simulink model "simu11"  (R2016b)
settings: Solver=VariableStepAuto  StartTime=0.0  StopTime=10.0  RelTol=1e-3
libraries: ArbolFallosLIB x185
settings Model: Creator=inmaculadacoronaperez  LastModifiedBy=josed

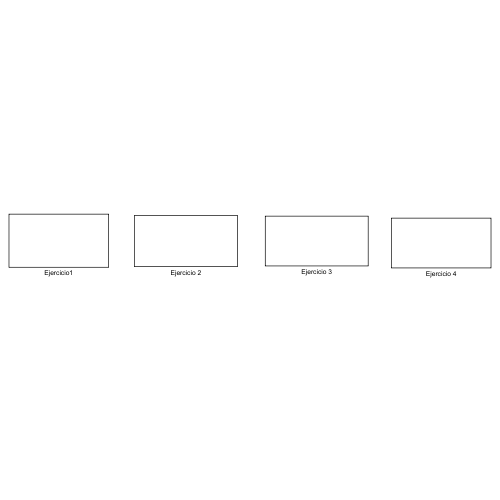
[thumbnail: Simulink's stored preview of the top-level diagram]
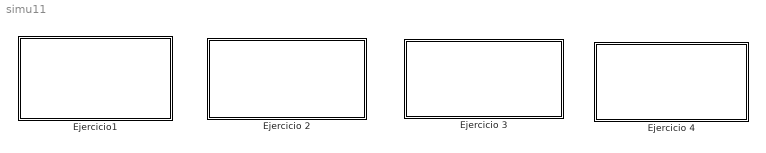
== system simu11 ==
  "Ejercicio 2 " : Subsystem
  "Ejercicio 3 " : Subsystem
  Ejercicio 4 : Subsystem
  "Ejercicio1 " : Subsystem

== system simu11/Ejercicio 2  ==
  Apartado b : Subsystem
  Apartado c : Subsystem
  wires:
  Apartado b/1(Out1) -> [s2_apb]
  [s2_apb] -> Apartado c/1(In1)

== system simu11/Ejercicio 3  ==
  APARTADO A : Subsystem
  Subsystem : Subsystem
  wires:
  APARTADO A/1(Out1) -> [lambda_elevador]
  [lambda_elevador] -> Subsystem/1(In1)

== system simu11/Ejercicio 4 ==
  APARTADO B : Subsystem
  APARTADO C : Subsystem
  APARTADO D : Subsystem
  APARTADO E : Subsystem

== system simu11/Ejercicio1  ==
  Ejercicio 1 a) : Subsystem
  Ejercicio 1 b) : Subsystem

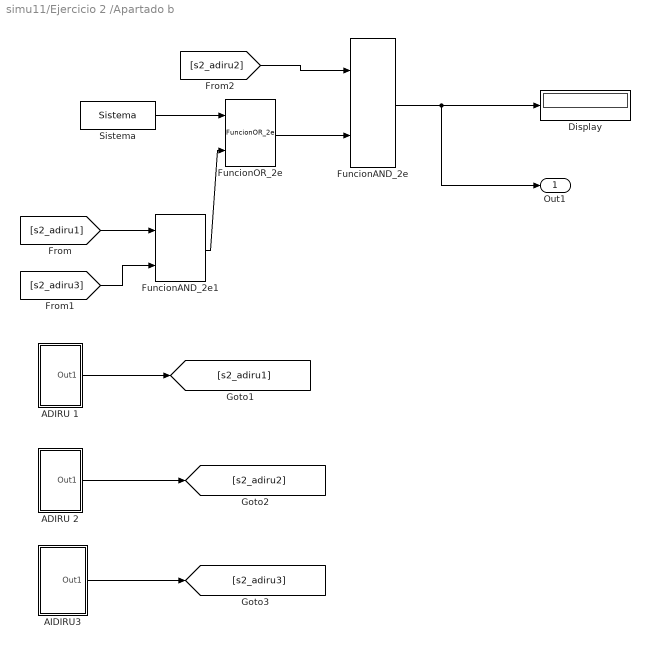
== system simu11/Ejercicio 2 /Apartado b ==
  ADIRU 1 : Subsystem
  ADIRU 2 : Subsystem
  AIDIRU3 : Subsystem
  Display : Display
  FuncionAND_2e : ArbolFallosLIB/FuncionAND_2e  SystemSampleTime=-1  Latency=0  AutoFrameSizeCalculation=off
  FuncionAND_2e1 : ArbolFallosLIB/FuncionAND_2e  SystemSampleTime=-1  Latency=0  AutoFrameSizeCalculation=off
  FuncionOR_2e : ArbolFallosLIB/FuncionOR_2e  SystemSampleTime=-1  Latency=0  AutoFrameSizeCalculation=off
  Sistema : ArbolFallosLIB/Sistema  sistema='CAPT TAT'  lambda=5e-04
  Out1 : Outport
  wires:
  [s2_adiru1] -> FuncionAND_2e1/1
  Sistema/1 -> FuncionOR_2e/1
  FuncionAND_2e/1 -> Out1/1, Display/1
  [s2_adiru3] -> FuncionAND_2e1/2
  FuncionAND_2e1/1 -> FuncionOR_2e/2
  FuncionOR_2e/1 -> FuncionAND_2e/2
  [s2_adiru2] -> FuncionAND_2e/1
  ADIRU 1/1(Out1) -> [s2_adiru1]
  ADIRU 2/1(Out1) -> [s2_adiru2]
  AIDIRU3/1(Out1) -> [s2_adiru3]

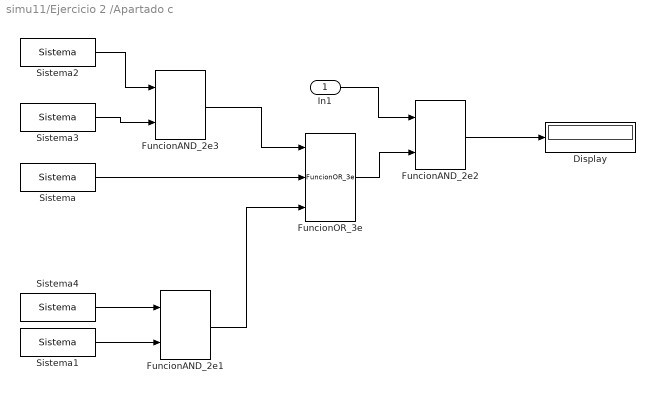
== system simu11/Ejercicio 2 /Apartado c ==
  In1 : Inport
  Display : Display
  FuncionAND_2e1 : ArbolFallosLIB/FuncionAND_2e  SystemSampleTime=-1  Latency=0  AutoFrameSizeCalculation=off
  FuncionAND_2e2 : ArbolFallosLIB/FuncionAND_2e  SystemSampleTime=-1  Latency=0  AutoFrameSizeCalculation=off
  FuncionAND_2e3 : ArbolFallosLIB/FuncionAND_2e  SystemSampleTime=-1  Latency=0  AutoFrameSizeCalculation=off
  FuncionOR_3e : ArbolFallosLIB/FuncionOR_3e  SystemSampleTime=-1  Latency=0  AutoFrameSizeCalculation=off
  Sistema : ArbolFallosLIB/Sistema  sistema='PITOT STBY'  lambda=2e-03
  Sistema1 : ArbolFallosLIB/Sistema  sistema='STATIC STBY'  lambda=1.5e-03
  Sistema2 : ArbolFallosLIB/Sistema  sistema='STBY ASI'  lambda=5e-03
  Sistema3 : ArbolFallosLIB/Sistema  sistema='STBY ALTI'  lambda=5e-03
  Sistema4 : ArbolFallosLIB/Sistema  sistema='STATIC STBY'  lambda=1.5e-03
  wires:
  Sistema/1 -> FuncionOR_3e/2
  Sistema4/1 -> FuncionAND_2e1/1
  Sistema1/1 -> FuncionAND_2e1/2
  FuncionAND_2e1/1 -> FuncionOR_3e/3
  FuncionOR_3e/1 -> FuncionAND_2e2/2
  Sistema2/1 -> FuncionAND_2e3/1
  Sistema3/1 -> FuncionAND_2e3/2
  FuncionAND_2e3/1 -> FuncionOR_3e/1
  In1/1 -> FuncionAND_2e2/1
  FuncionAND_2e2/1 -> Display/1

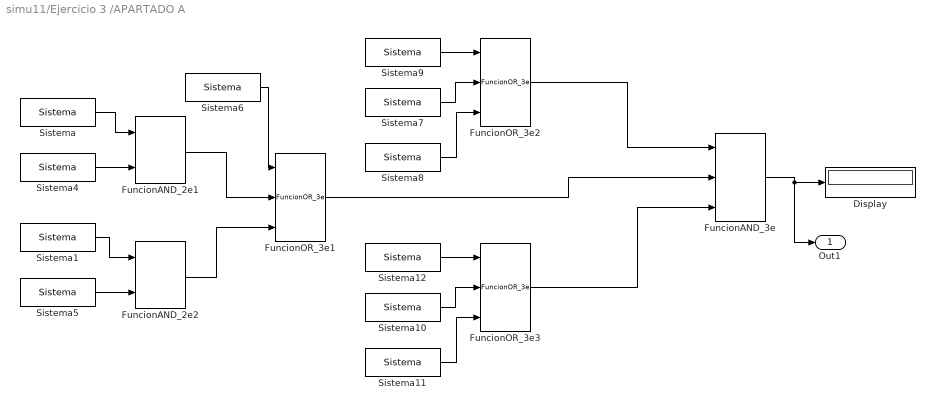
== system simu11/Ejercicio 3 /APARTADO A ==
  Display : Display
  FuncionAND_2e1 : ArbolFallosLIB/FuncionAND_2e  SystemSampleTime=-1  Latency=0  AutoFrameSizeCalculation=off
  FuncionAND_2e2 : ArbolFallosLIB/FuncionAND_2e  SystemSampleTime=-1  Latency=0  AutoFrameSizeCalculation=off
  FuncionAND_3e : ArbolFallosLIB/FuncionAND_3e  SystemSampleTime=-1  Latency=0  AutoFrameSizeCalculation=off
  FuncionOR_3e1 : ArbolFallosLIB/FuncionOR_3e  SystemSampleTime=-1  Latency=0  AutoFrameSizeCalculation=off
  FuncionOR_3e2 : ArbolFallosLIB/FuncionOR_3e  SystemSampleTime=-1  Latency=0  AutoFrameSizeCalculation=off
  FuncionOR_3e3 : ArbolFallosLIB/FuncionOR_3e  SystemSampleTime=-1  Latency=0  AutoFrameSizeCalculation=off
  Sistema : ArbolFallosLIB/Sistema  sistema='ACT RHO'  lambda=2.5e-04
  Sistema1 : ArbolFallosLIB/Sistema  sistema='Databus 2'  lambda=1e-8
  Sistema10 : ArbolFallosLIB/Sistema  sistema='HYD G'  lambda=2e-4
  Sistema11 : ArbolFallosLIB/Sistema  sistema='Databus 4'  lambda=1e-8
  Sistema12 : ArbolFallosLIB/Sistema  sistema='ACTUADOR LHI'  lambda=2.5e-04
  Sistema4 : ArbolFallosLIB/Sistema  sistema='ACT LHO'  lambda=2.5e-04
  Sistema5 : ArbolFallosLIB/Sistema  sistema='Databus 3'  lambda=1e-8
  Sistema6 : ArbolFallosLIB/Sistema  sistema='HYD B'  lambda=2e-4
  Sistema7 : ArbolFallosLIB/Sistema  sistema='HYD Y'  lambda=2e-4
  Sistema8 : ArbolFallosLIB/Sistema  sistema='Databus 1'  lambda=1e-8
  Sistema9 : ArbolFallosLIB/Sistema  sistema='ACTUADOR RHI'  lambda=2.5e-04
  Out1 : Outport
  wires:
  FuncionAND_3e/1 -> Display/1, Out1/1
  FuncionAND_2e2/1 -> FuncionOR_3e1/3
  Sistema5/1 -> FuncionAND_2e2/2
  Sistema9/1 -> FuncionOR_3e2/1
  Sistema/1 -> FuncionAND_2e1/1
  Sistema4/1 -> FuncionAND_2e1/2
  Sistema8/1 -> FuncionOR_3e2/3
  FuncionOR_3e3/1 -> FuncionAND_3e/3
  Sistema7/1 -> FuncionOR_3e2/2
  FuncionOR_3e2/1 -> FuncionAND_3e/1
  Sistema12/1 -> FuncionOR_3e3/1
  Sistema10/1 -> FuncionOR_3e3/2
  Sistema11/1 -> FuncionOR_3e3/3
  FuncionOR_3e1/1 -> FuncionAND_3e/2
  FuncionAND_2e1/1 -> FuncionOR_3e1/2
  Sistema1/1 -> FuncionAND_2e2/1
  Sistema6/1 -> FuncionOR_3e1/1

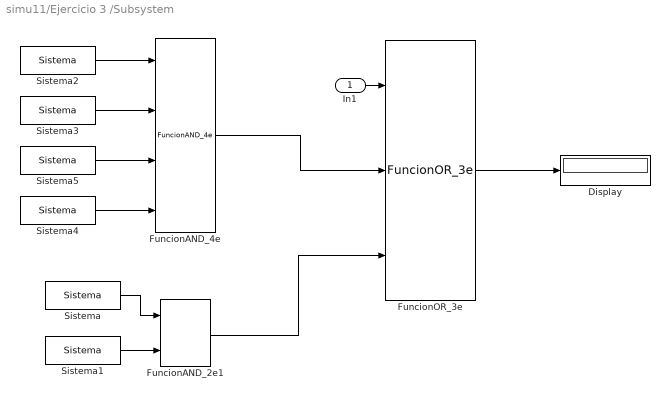
== system simu11/Ejercicio 3 /Subsystem ==
  In1 : Inport
  Display : Display
  FuncionAND_2e1 : ArbolFallosLIB/FuncionAND_2e  SystemSampleTime=-1  Latency=0  AutoFrameSizeCalculation=off
  FuncionAND_4e : ArbolFallosLIB/FuncionAND_4e  SystemSampleTime=-1  Latency=0  AutoFrameSizeCalculation=off
  FuncionOR_3e : ArbolFallosLIB/FuncionOR_3e  SystemSampleTime=-1  Latency=0  AutoFrameSizeCalculation=off
  Sistema : ArbolFallosLIB/Sistema  sistema='STICK CAPT'  lambda=2e-06
  Sistema1 : ArbolFallosLIB/Sistema  sistema='STICK F/O'  lambda=2e-06
  Sistema2 : ArbolFallosLIB/Sistema  sistema='ELAC 1'  lambda=1e-04
  Sistema3 : ArbolFallosLIB/Sistema  sistema='ELAC 2'  lambda=1e-04
  Sistema4 : ArbolFallosLIB/Sistema  sistema='ELAC 4'  lambda=1e-04
  Sistema5 : ArbolFallosLIB/Sistema  sistema='ELAC 3'  lambda=1e-04
  wires:
  Sistema3/1 -> FuncionAND_4e/2
  Sistema/1 -> FuncionAND_2e1/1
  FuncionAND_2e1/1 -> FuncionOR_3e/3
  Sistema1/1 -> FuncionAND_2e1/2
  Sistema4/1 -> FuncionAND_4e/4
  Sistema2/1 -> FuncionAND_4e/1
  FuncionAND_4e/1 -> FuncionOR_3e/2
  In1/1 -> FuncionOR_3e/1
  Sistema5/1 -> FuncionAND_4e/3
  FuncionOR_3e/1 -> Display/1

== system simu11/Ejercicio 4/APARTADO B ==
  Display : Display
  FuncionOR_2e1 : ArbolFallosLIB/FuncionOR_2e  SystemSampleTime=-1  Latency=0  AutoFrameSizeCalculation=off
  FuncionOR_2e2 : ArbolFallosLIB/FuncionOR_2e  SystemSampleTime=-1  Latency=0  AutoFrameSizeCalculation=off
  FuncionOR_2e3 : ArbolFallosLIB/FuncionOR_2e  SystemSampleTime=-1  Latency=0  AutoFrameSizeCalculation=off
  Sistema : ArbolFallosLIB/Sistema  sistema='COM'  lambda=5e-4
  Sistema1 : ArbolFallosLIB/Sistema  sistema='MON'  lambda=7e-4
  Sistema2 : ArbolFallosLIB/Sistema  sistema='COM'  lambda=5e-4
  Sistema3 : ArbolFallosLIB/Sistema  sistema='MON'  lambda=7e-4
  wires:
  FuncionOR_2e3/1 -> Display/1
  Sistema1/1 -> FuncionOR_2e1/2
  Sistema/1 -> FuncionOR_2e1/1
  Sistema3/1 -> FuncionOR_2e2/2
  Sistema2/1 -> FuncionOR_2e2/1
  FuncionOR_2e1/1 -> FuncionOR_2e3/1
  FuncionOR_2e2/1 -> FuncionOR_2e3/2

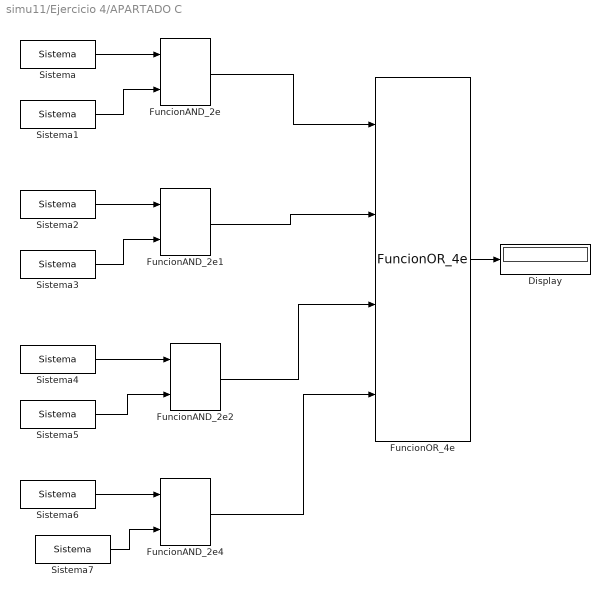
== system simu11/Ejercicio 4/APARTADO C ==
  Display : Display
  FuncionAND_2e{,1..2,4} (4 alike) : ArbolFallosLIB/FuncionAND_2e  SystemSampleTime=-1  Latency=0  AutoFrameSizeCalculation=off
  FuncionOR_4e : ArbolFallosLIB/FuncionOR_4e  SystemSampleTime=-1  Latency=0  AutoFrameSizeCalculation=off
  Sistema : ArbolFallosLIB/Sistema  sistema='COM_A'  lambda=5e-4
  Sistema1 : ArbolFallosLIB/Sistema  sistema='COM_B'  lambda=5e-4
  Sistema2 : ArbolFallosLIB/Sistema  sistema='MON_A'  lambda=7e-4
  Sistema3 : ArbolFallosLIB/Sistema  sistema='MON_B'  lambda=7e-4
  Sistema4 : ArbolFallosLIB/Sistema  sistema='COM_A'  lambda=5e-4
  Sistema5 : ArbolFallosLIB/Sistema  sistema='MON_B'  lambda=7e-4
  Sistema6 : ArbolFallosLIB/Sistema  sistema='MON_A'  lambda=7e-4
  Sistema7 : ArbolFallosLIB/Sistema  sistema='COM_B'  lambda=5e-4
  wires:
  Sistema1/1 -> FuncionAND_2e/2
  Sistema/1 -> FuncionAND_2e/1
  Sistema6/1 -> FuncionAND_2e4/1
  Sistema7/1 -> FuncionAND_2e4/2
  FuncionAND_2e1/1 -> FuncionOR_4e/2
  FuncionAND_2e4/1 -> FuncionOR_4e/4
  Sistema5/1 -> FuncionAND_2e2/2
  Sistema2/1 -> FuncionAND_2e1/1
  Sistema3/1 -> FuncionAND_2e1/2
  FuncionAND_2e/1 -> FuncionOR_4e/1
  FuncionOR_4e/1 -> Display/1
  Sistema4/1 -> FuncionAND_2e2/1
  FuncionAND_2e2/1 -> FuncionOR_4e/3

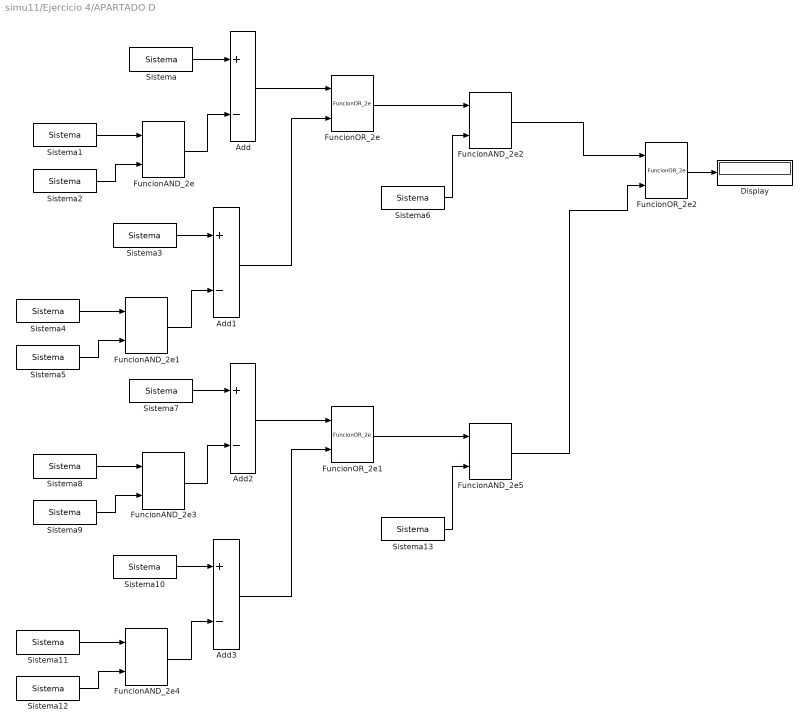
== system simu11/Ejercicio 4/APARTADO D ==
  Add{,1..3} (4 alike) : Sum  Inputs=+-
  Display : Display
  FuncionAND_2e{,1..5} (6 alike) : ArbolFallosLIB/FuncionAND_2e  SystemSampleTime=-1  Latency=0  AutoFrameSizeCalculation=off
  FuncionOR_2e : ArbolFallosLIB/FuncionOR_2e  SystemSampleTime=-1  Latency=0  AutoFrameSizeCalculation=off
  FuncionOR_2e1 : ArbolFallosLIB/FuncionOR_2e  SystemSampleTime=-1  Latency=0  AutoFrameSizeCalculation=off
  FuncionOR_2e2 : ArbolFallosLIB/FuncionOR_2e  SystemSampleTime=-1  Latency=0  AutoFrameSizeCalculation=off
  Sistema{,1,7..8} (4 alike) : ArbolFallosLIB/Sistema  sistema='COM'  lambda=5e-4
  Sistema{3..4,10..11} (4 alike) : ArbolFallosLIB/Sistema  sistema='MON'  lambda=7e-4
  Sistema{2,5,9,12} (4 alike) : ArbolFallosLIB/Sistema  sistema='BIT'  lambda=0.92
  Sistema13 : ArbolFallosLIB/Sistema  sistema='XMON'  lambda=0.04
  Sistema6 : ArbolFallosLIB/Sistema  sistema='XMON'  lambda=0.04
  wires:
  FuncionOR_2e/1 -> FuncionAND_2e2/1
  Sistema6/1 -> FuncionAND_2e2/2
  Sistema1/1 -> FuncionAND_2e/1
  Sistema2/1 -> FuncionAND_2e/2
  FuncionAND_2e2/1 -> FuncionOR_2e2/1
  FuncionAND_2e/1 -> Add/2
  Add1/1 -> FuncionOR_2e/2
  Sistema7/1 -> Add2/1
  FuncionAND_2e3/1 -> Add2/2
  Sistema8/1 -> FuncionAND_2e3/1
  Sistema9/1 -> FuncionAND_2e3/2
  Add2/1 -> FuncionOR_2e1/1
  Sistema10/1 -> Add3/1
  FuncionAND_2e4/1 -> Add3/2
  Sistema11/1 -> FuncionAND_2e4/1
  Sistema12/1 -> FuncionAND_2e4/2
  Add3/1 -> FuncionOR_2e1/2
  FuncionOR_2e1/1 -> FuncionAND_2e5/1
  Sistema13/1 -> FuncionAND_2e5/2
  Sistema/1 -> Add/1
  Add/1 -> FuncionOR_2e/1
  FuncionOR_2e2/1 -> Display/1
  FuncionAND_2e5/1 -> FuncionOR_2e2/2
  Sistema3/1 -> Add1/1
  FuncionAND_2e1/1 -> Add1/2
  Sistema4/1 -> FuncionAND_2e1/1
  Sistema5/1 -> FuncionAND_2e1/2

== system simu11/Ejercicio 4/APARTADO E ==
  Display : Display
  FuncionAND_2e : ArbolFallosLIB/FuncionAND_2e  SystemSampleTime=-1  Latency=0  AutoFrameSizeCalculation=off
  FuncionAND_2e1 : ArbolFallosLIB/FuncionAND_2e  SystemSampleTime=-1  Latency=0  AutoFrameSizeCalculation=off
  FuncionOR_2e : ArbolFallosLIB/FuncionOR_2e  SystemSampleTime=-1  Latency=0  AutoFrameSizeCalculation=off
  Sistema : ArbolFallosLIB/Sistema  sistema='COM_A'  lambda=5e-4
  Sistema1 : ArbolFallosLIB/Sistema  sistema='COM_B'  lambda=5e-4
  Sistema2 : ArbolFallosLIB/Sistema  sistema='MON_A'  lambda=7e-4
  Sistema3 : ArbolFallosLIB/Sistema  sistema='MON_B'  lambda=7e-4
  wires:
  FuncionAND_2e1/1 -> FuncionOR_2e/2
  Sistema/1 -> FuncionAND_2e/1
  FuncionOR_2e/1 -> Display/1
  Sistema1/1 -> FuncionAND_2e1/1
  Sistema3/1 -> FuncionAND_2e1/2
  Sistema2/1 -> FuncionAND_2e/2
  FuncionAND_2e/1 -> FuncionOR_2e/1

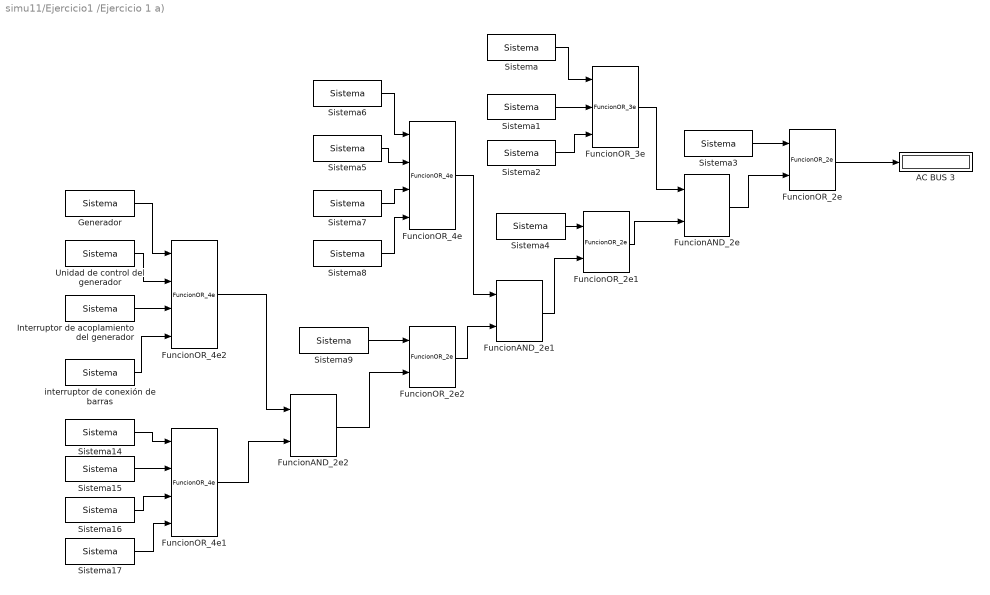
== system simu11/Ejercicio1 /Ejercicio 1 a) ==
  AC BUS 3 : Display
  FuncionAND_2e : ArbolFallosLIB/FuncionAND_2e  SystemSampleTime=-1  Latency=0  AutoFrameSizeCalculation=off
  FuncionAND_2e1 : ArbolFallosLIB/FuncionAND_2e  SystemSampleTime=-1  Latency=0  AutoFrameSizeCalculation=off
  FuncionAND_2e2 : ArbolFallosLIB/FuncionAND_2e  SystemSampleTime=-1  Latency=0  AutoFrameSizeCalculation=off
  FuncionOR_2e : ArbolFallosLIB/FuncionOR_2e  SystemSampleTime=-1  Latency=0  AutoFrameSizeCalculation=off
  FuncionOR_2e1 : ArbolFallosLIB/FuncionOR_2e  SystemSampleTime=-1  Latency=0  AutoFrameSizeCalculation=off
  FuncionOR_2e2 : ArbolFallosLIB/FuncionOR_2e  SystemSampleTime=-1  Latency=0  AutoFrameSizeCalculation=off
  FuncionOR_3e : ArbolFallosLIB/FuncionOR_3e  SystemSampleTime=-1  Latency=0  AutoFrameSizeCalculation=off
  FuncionOR_4e : ArbolFallosLIB/FuncionOR_4e  SystemSampleTime=-1  Latency=0  AutoFrameSizeCalculation=off
  FuncionOR_4e1 : ArbolFallosLIB/FuncionOR_4e  SystemSampleTime=-1  Latency=0  AutoFrameSizeCalculation=off
  FuncionOR_4e2 : ArbolFallosLIB/FuncionOR_4e  SystemSampleTime=-1  Latency=0  AutoFrameSizeCalculation=off
  Generador : ArbolFallosLIB/Sistema  sistema='IDG 1'  lambda=4e-4
  Interruptor de acoplamiento del generador : ArbolFallosLIB/Sistema  sistema='GCB 1'  lambda=1.5e-4
  Sistema : ArbolFallosLIB/Sistema  sistema='IDG 3'  lambda=4e-4
  Sistema1 : ArbolFallosLIB/Sistema  sistema='GCU 3'  lambda=3e-4
  Sistema14 : ArbolFallosLIB/Sistema  sistema='IDG 2'  lambda=4e-4
  Sistema15 : ArbolFallosLIB/Sistema  sistema='GCU 2'  lambda=3e-4
  Sistema16 : ArbolFallosLIB/Sistema  sistema='GCB 2'  lambda=1.5e-4
  Sistema17 : ArbolFallosLIB/Sistema  sistema='BTB 2'  lambda=1.5e-4
  Sistema2 : ArbolFallosLIB/Sistema  sistema='GCB 3'  lambda=1.5e-4
  Sistema3 : ArbolFallosLIB/Sistema  sistema='ELCU'  lambda=3.5e-4
  Sistema4 : ArbolFallosLIB/Sistema  sistema='BTB 3'  lambda=1.5e-4
  Sistema5 : ArbolFallosLIB/Sistema  sistema='GCU 4'  lambda=3e-4
  Sistema6 : ArbolFallosLIB/Sistema  sistema='IDG 4'  lambda=4e-4
  Sistema7 : ArbolFallosLIB/Sistema  sistema='GCB 4'  lambda=1.5e-4
  Sistema8 : ArbolFallosLIB/Sistema  sistema='BTB 4'  lambda=1.5e-4
  Sistema9 : ArbolFallosLIB/Sistema  sistema='SSB'  lambda=1.5e-4
  Unidad de control del generador : ArbolFallosLIB/Sistema  sistema='GCU 1'  lambda=3e-4
  interruptor de conexión de barras : ArbolFallosLIB/Sistema  sistema='BTB 1'  lambda=1.5e-4
  wires:
  FuncionOR_2e/1 -> AC BUS 3/1
  FuncionOR_2e2/1 -> FuncionAND_2e1/2
  interruptor de conexión de barras/1 -> FuncionOR_4e2/4
  FuncionAND_2e1/1 -> FuncionOR_2e1/2
  Sistema4/1 -> FuncionOR_2e1/1
  Sistema6/1 -> FuncionOR_4e/1
  Sistema2/1 -> FuncionOR_3e/3
  Sistema17/1 -> FuncionOR_4e1/4
  FuncionAND_2e2/1 -> FuncionOR_2e2/2
  FuncionOR_4e1/1 -> FuncionAND_2e2/2
  Sistema16/1 -> FuncionOR_4e1/3
  Generador/1 -> FuncionOR_4e2/1
  FuncionOR_2e1/1 -> FuncionAND_2e/2
  FuncionOR_4e2/1 -> FuncionAND_2e2/1
  Sistema5/1 -> FuncionOR_4e/2
  Sistema15/1 -> FuncionOR_4e1/2
  Sistema7/1 -> FuncionOR_4e/3
  Sistema8/1 -> FuncionOR_4e/4
  Sistema14/1 -> FuncionOR_4e1/1
  Interruptor de acoplamiento del generador/1 -> FuncionOR_4e2/3
  Sistema9/1 -> FuncionOR_2e2/1
  Sistema/1 -> FuncionOR_3e/1
  Unidad de control del generador/1 -> FuncionOR_4e2/2
  FuncionOR_3e/1 -> FuncionAND_2e/1
  FuncionAND_2e/1 -> FuncionOR_2e/2
  Sistema3/1 -> FuncionOR_2e/1
  Sistema1/1 -> FuncionOR_3e/2
  FuncionOR_4e/1 -> FuncionAND_2e1/1

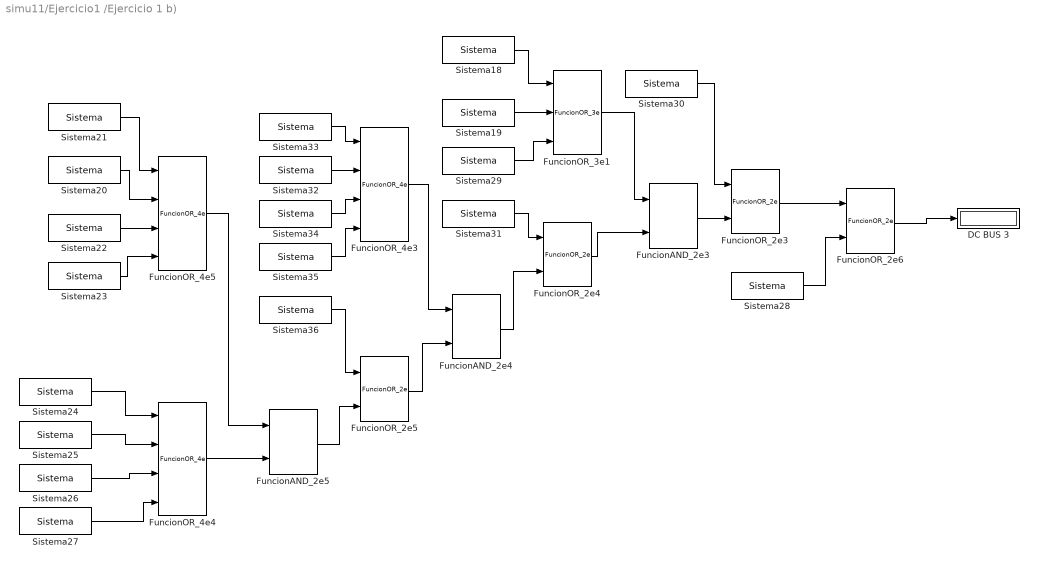
== system simu11/Ejercicio1 /Ejercicio 1 b) ==
  DC BUS 3 : Display
  FuncionAND_2e3 : ArbolFallosLIB/FuncionAND_2e  SystemSampleTime=-1  Latency=0  AutoFrameSizeCalculation=off
  FuncionAND_2e4 : ArbolFallosLIB/FuncionAND_2e  SystemSampleTime=-1  Latency=0  AutoFrameSizeCalculation=off
  FuncionAND_2e5 : ArbolFallosLIB/FuncionAND_2e  SystemSampleTime=-1  Latency=0  AutoFrameSizeCalculation=off
  FuncionOR_2e{3..6} (4 alike) : ArbolFallosLIB/FuncionOR_2e  SystemSampleTime=-1  Latency=0  AutoFrameSizeCalculation=off
  FuncionOR_3e1 : ArbolFallosLIB/FuncionOR_3e  SystemSampleTime=-1  Latency=0  AutoFrameSizeCalculation=off
  FuncionOR_4e3 : ArbolFallosLIB/FuncionOR_4e  SystemSampleTime=-1  Latency=0  AutoFrameSizeCalculation=off
  FuncionOR_4e4 : ArbolFallosLIB/FuncionOR_4e  SystemSampleTime=-1  Latency=0  AutoFrameSizeCalculation=off
  FuncionOR_4e5 : ArbolFallosLIB/FuncionOR_4e  SystemSampleTime=-1  Latency=0  AutoFrameSizeCalculation=off
  Sistema18 : ArbolFallosLIB/Sistema  sistema='IDG 3'  lambda=4e-4
  Sistema19 : ArbolFallosLIB/Sistema  sistema='GCU 3'  lambda=3e-4
  Sistema20 : ArbolFallosLIB/Sistema  sistema='GCU 1'  lambda=3e-4
  Sistema21 : ArbolFallosLIB/Sistema  sistema='IDG 1'  lambda=4e-4
  Sistema22 : ArbolFallosLIB/Sistema  sistema='GCB 1'  lambda=1.5e-4
  Sistema23 : ArbolFallosLIB/Sistema  sistema='BTB 1'  lambda=1.5e-4
  Sistema24 : ArbolFallosLIB/Sistema  sistema='IDG 2'  lambda=4e-4
  Sistema25 : ArbolFallosLIB/Sistema  sistema='GCU 2'  lambda=3e-4
  Sistema26 : ArbolFallosLIB/Sistema  sistema='GCB 2'  lambda=1.5e-4
  Sistema27 : ArbolFallosLIB/Sistema  sistema='BTB 2'  lambda=1.5e-4
  Sistema28 : ArbolFallosLIB/Sistema  sistema='TRU 3'  lambda=5e-4
  Sistema29 : ArbolFallosLIB/Sistema  sistema='GCB 3'  lambda=1.5e-4
  Sistema30 : ArbolFallosLIB/Sistema  sistema='ELCU'  lambda=3.5e-4
  Sistema31 : ArbolFallosLIB/Sistema  sistema='BTB 3'  lambda=1.5e-4
  Sistema32 : ArbolFallosLIB/Sistema  sistema='GCU 4'  lambda=3e-4
  Sistema33 : ArbolFallosLIB/Sistema  sistema='IDG 4'  lambda=4e-4
  Sistema34 : ArbolFallosLIB/Sistema  sistema='GCB 4'  lambda=1.5e-4
  Sistema35 : ArbolFallosLIB/Sistema  sistema='BTB 4'  lambda=1.5e-4
  Sistema36 : ArbolFallosLIB/Sistema  sistema='SSB'  lambda=1.5e-4
  wires:
  Sistema33/1 -> FuncionOR_4e3/1
  Sistema29/1 -> FuncionOR_3e1/3
  Sistema26/1 -> FuncionOR_4e4/3
  Sistema35/1 -> FuncionOR_4e3/4
  FuncionAND_2e3/1 -> FuncionOR_2e3/2
  FuncionAND_2e5/1 -> FuncionOR_2e5/2
  Sistema20/1 -> FuncionOR_4e5/2
  FuncionOR_2e5/1 -> FuncionAND_2e4/2
  Sistema24/1 -> FuncionOR_4e4/1
  FuncionOR_2e3/1 -> FuncionOR_2e6/1
  FuncionOR_2e6/1 -> DC BUS 3/1
  Sistema22/1 -> FuncionOR_4e5/3
  Sistema32/1 -> FuncionOR_4e3/2
  Sistema28/1 -> FuncionOR_2e6/2
  Sistema25/1 -> FuncionOR_4e4/2
  Sistema18/1 -> FuncionOR_3e1/1
  FuncionOR_4e5/1 -> FuncionAND_2e5/1
  FuncionOR_3e1/1 -> FuncionAND_2e3/1
  Sistema27/1 -> FuncionOR_4e4/4
  Sistema19/1 -> FuncionOR_3e1/2
  FuncionOR_4e3/1 -> FuncionAND_2e4/1
  FuncionOR_4e4/1 -> FuncionAND_2e5/2
  Sistema34/1 -> FuncionOR_4e3/3
  FuncionOR_2e4/1 -> FuncionAND_2e3/2
  Sistema31/1 -> FuncionOR_2e4/1
  Sistema36/1 -> FuncionOR_2e5/1
  Sistema30/1 -> FuncionOR_2e3/1
  Sistema23/1 -> FuncionOR_4e5/4
  Sistema21/1 -> FuncionOR_4e5/1
  FuncionAND_2e4/1 -> FuncionOR_2e4/2

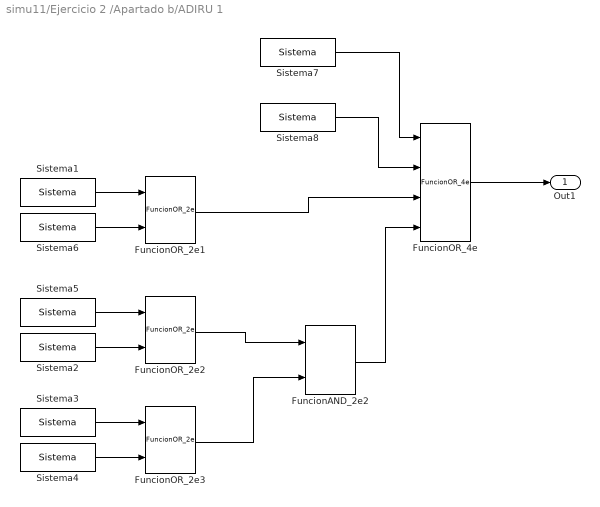
== system simu11/Ejercicio 2 /Apartado b/ADIRU 1 ==
  FuncionAND_2e2 : ArbolFallosLIB/FuncionAND_2e  SystemSampleTime=-1  Latency=0  AutoFrameSizeCalculation=off
  FuncionOR_2e1 : ArbolFallosLIB/FuncionOR_2e  SystemSampleTime=-1  Latency=0  AutoFrameSizeCalculation=off
  FuncionOR_2e2 : ArbolFallosLIB/FuncionOR_2e  SystemSampleTime=-1  Latency=0  AutoFrameSizeCalculation=off
  FuncionOR_2e3 : ArbolFallosLIB/FuncionOR_2e  SystemSampleTime=-1  Latency=0  AutoFrameSizeCalculation=off
  FuncionOR_4e : ArbolFallosLIB/FuncionOR_4e  SystemSampleTime=-1  Latency=0  AutoFrameSizeCalculation=off
  Sistema1 : ArbolFallosLIB/Sistema  sistema='PITOT CAPT'  lambda=2e-03
  Sistema2 : ArbolFallosLIB/Sistema  sistema='ADM'  lambda=1e-04
  Sistema3 : ArbolFallosLIB/Sistema  sistema='STATIC CAPT'  lambda=1.5e-04
  Sistema4 : ArbolFallosLIB/Sistema  sistema='ADM'  lambda=1e-04
  Sistema5 : ArbolFallosLIB/Sistema  sistema='STATIC CAPT'  lambda=1.5e-04
  Sistema6 : ArbolFallosLIB/Sistema  sistema='ADM'  lambda=1e-04
  Sistema7 : ArbolFallosLIB/Sistema  sistema='ADIRU 1'  lambda=2.5e-04
  Sistema8 : ArbolFallosLIB/Sistema  sistema='CAPT AOA'  lambda=7.5e-03
  Out1 : Outport
  wires:
  Sistema4/1 -> FuncionOR_2e3/2
  Sistema3/1 -> FuncionOR_2e3/1
  FuncionOR_2e2/1 -> FuncionAND_2e2/1
  Sistema2/1 -> FuncionOR_2e2/2
  FuncionOR_2e3/1 -> FuncionAND_2e2/2
  Sistema1/1 -> FuncionOR_2e1/1
  Sistema8/1 -> FuncionOR_4e/2
  Sistema6/1 -> FuncionOR_2e1/2
  FuncionOR_4e/1 -> Out1/1
  Sistema5/1 -> FuncionOR_2e2/1
  FuncionOR_2e1/1 -> FuncionOR_4e/3
  FuncionAND_2e2/1 -> FuncionOR_4e/4
  Sistema7/1 -> FuncionOR_4e/1

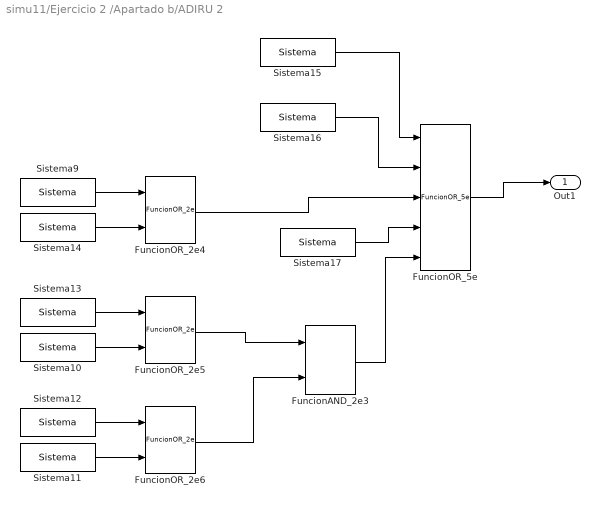
== system simu11/Ejercicio 2 /Apartado b/ADIRU 2 ==
  FuncionAND_2e3 : ArbolFallosLIB/FuncionAND_2e  SystemSampleTime=-1  Latency=0  AutoFrameSizeCalculation=off
  FuncionOR_2e4 : ArbolFallosLIB/FuncionOR_2e  SystemSampleTime=-1  Latency=0  AutoFrameSizeCalculation=off
  FuncionOR_2e5 : ArbolFallosLIB/FuncionOR_2e  SystemSampleTime=-1  Latency=0  AutoFrameSizeCalculation=off
  FuncionOR_2e6 : ArbolFallosLIB/FuncionOR_2e  SystemSampleTime=-1  Latency=0  AutoFrameSizeCalculation=off
  FuncionOR_5e : ArbolFallosLIB/FuncionOR_5e  SystemSampleTime=-1  Latency=0  AutoFrameSizeCalculation=off
  Sistema10 : ArbolFallosLIB/Sistema  sistema='ADM'  lambda=1e-04
  Sistema11 : ArbolFallosLIB/Sistema  sistema='STATIC F/O'  lambda=1.5e-04
  Sistema12 : ArbolFallosLIB/Sistema  sistema='ADM'  lambda=1e-04
  Sistema13 : ArbolFallosLIB/Sistema  sistema='STATIC F/O'  lambda=1.5e-04
  Sistema14 : ArbolFallosLIB/Sistema  sistema='ADM'  lambda=1e-04
  Sistema15 : ArbolFallosLIB/Sistema  sistema='ADIRU 2'  lambda=2.5e-04
  Sistema16 : ArbolFallosLIB/Sistema  sistema='F/O AOA'  lambda=7.5e-03
  Sistema17 : ArbolFallosLIB/Sistema  sistema='F/O TAT'  lambda=5e-04
  Sistema9 : ArbolFallosLIB/Sistema  sistema='PITOT F/O'  lambda=2e-03
  Out1 : Outport
  wires:
  FuncionOR_2e5/1 -> FuncionAND_2e3/1
  Sistema10/1 -> FuncionOR_2e5/2
  FuncionOR_2e6/1 -> FuncionAND_2e3/2
  Sistema9/1 -> FuncionOR_2e4/1
  Sistema16/1 -> FuncionOR_5e/2
  Sistema14/1 -> FuncionOR_2e4/2
  Sistema13/1 -> FuncionOR_2e5/1
  FuncionOR_2e4/1 -> FuncionOR_5e/3
  Sistema15/1 -> FuncionOR_5e/1
  Sistema12/1 -> FuncionOR_2e6/1
  Sistema11/1 -> FuncionOR_2e6/2
  FuncionAND_2e3/1 -> FuncionOR_5e/5
  Sistema17/1 -> FuncionOR_5e/4
  FuncionOR_5e/1 -> Out1/1

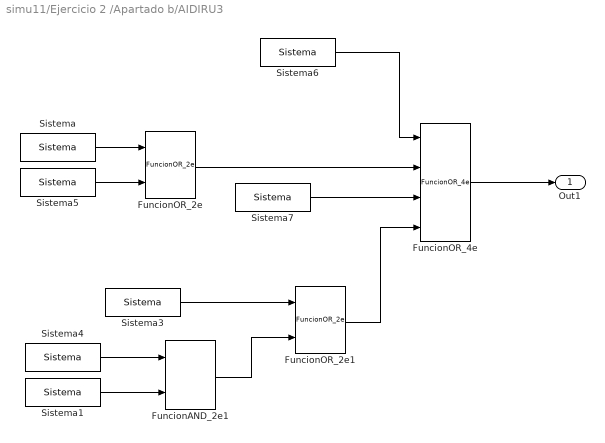
== system simu11/Ejercicio 2 /Apartado b/AIDIRU3 ==
  FuncionAND_2e1 : ArbolFallosLIB/FuncionAND_2e  SystemSampleTime=-1  Latency=0  AutoFrameSizeCalculation=off
  FuncionOR_2e : ArbolFallosLIB/FuncionOR_2e  SystemSampleTime=-1  Latency=0  AutoFrameSizeCalculation=off
  FuncionOR_2e1 : ArbolFallosLIB/FuncionOR_2e  SystemSampleTime=-1  Latency=0  AutoFrameSizeCalculation=off
  FuncionOR_4e : ArbolFallosLIB/FuncionOR_4e  SystemSampleTime=-1  Latency=0  AutoFrameSizeCalculation=off
  Sistema : ArbolFallosLIB/Sistema  sistema='PITOT STBY'  lambda=2e-03
  Sistema1 : ArbolFallosLIB/Sistema  sistema='STATIC STBY'  lambda=1.5e-04
  Sistema3 : ArbolFallosLIB/Sistema  sistema='ADM'  lambda=1e-04
  Sistema4 : ArbolFallosLIB/Sistema  sistema='STATIC STBY'  lambda=1.5e-04
  Sistema5 : ArbolFallosLIB/Sistema  sistema='ADM'  lambda=1e-04
  Sistema6 : ArbolFallosLIB/Sistema  sistema='ADIRU 3'  lambda=2.5e-04
  Sistema7 : ArbolFallosLIB/Sistema  sistema='STBY AOA'  lambda=7.5e-03
  Out1 : Outport
  wires:
  Sistema/1 -> FuncionOR_2e/1
  Sistema5/1 -> FuncionOR_2e/2
  Sistema6/1 -> FuncionOR_4e/1
  FuncionOR_2e/1 -> FuncionOR_4e/2
  Sistema7/1 -> FuncionOR_4e/3
  Sistema4/1 -> FuncionAND_2e1/1
  Sistema1/1 -> FuncionAND_2e1/2
  Sistema3/1 -> FuncionOR_2e1/1
  FuncionAND_2e1/1 -> FuncionOR_2e1/2
  FuncionOR_2e1/1 -> FuncionOR_4e/4
  FuncionOR_4e/1 -> Out1/1
